simulink model "guidance_formationBreak"  (R2023a)
settings: Solver=ode4  StartTime=0.0  StopTime=10.0  FixedStep=dt  RelTol=1e-3
undefined symbols (not defined in the file): dt, gnc
settings Model: Creator=hugobuurmeijer  LastModifiedBy=hugobuurmeijer

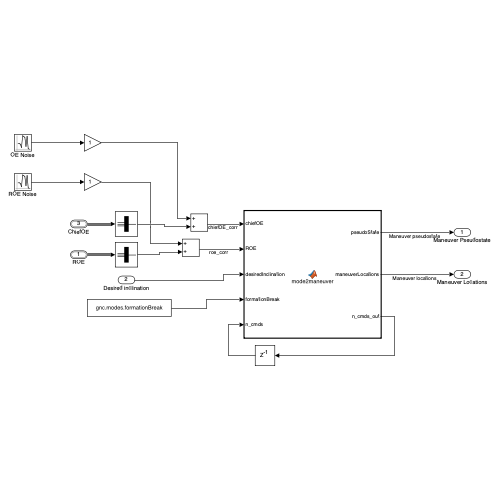
[thumbnail: Simulink's stored preview of the top-level diagram]
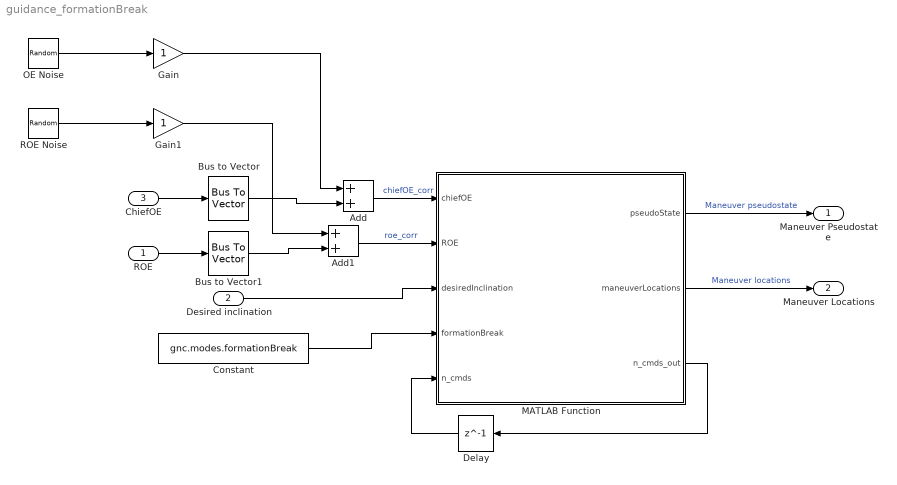
== system guidance_formationBreak ==
  ROE : Inport  OutDataTypeStr=Bus: eccentricSingularROE
  Desired inclination : Inport  Port=2  PortDimensions=2
  ChiefOE : Inport  Port=3  OutDataTypeStr=Bus: meanOrbitElements
  Add : Sum
  Add1 : Sum
  Bus to Vector : BusToVector
  Bus to Vector1 : BusToVector
  Constant : Constant  Value=gnc.modes.formationBreak
  Delay : Delay  DelayLength=1  InitialCondition=0
  Gain : Gain
  Gain1 : Gain
  MATLAB Function : MATLAB Function  TreatAsAtomicUnit=on
  OE Noise : RandomNumber  Mean=zeros(6,1)  Variance=[100,1e-6,1e-6,1e-6,1e-6,1e-46]'  Seed=[1;2;3;4;5;6]  SampleTime=dt
  ROE Noise : RandomNumber  Mean=zeros(6,1)  Variance=1e-12*ones(6,1)  Seed=[1;2;3;4;5;6]  SampleTime=dt
  Maneuver Pseudostate : Outport
  Maneuver Locations : Outport  Port=2
  wires:
  ROE/1 -> Bus to Vector1/1
  Desired inclination/1 -> MATLAB Function/3(desiredInclination)
  MATLAB Function/1(pseudoState) -> Maneuver Pseudostate/1  "Maneuver pseudostate"
  MATLAB Function/2(maneuverLocations) -> Maneuver Locations/1  "Maneuver locations"
  ChiefOE/1 -> Bus to Vector/1
  Bus to Vector/1 -> Add/2
  Bus to Vector1/1 -> Add1/2
  MATLAB Function/3(n_cmds_out) -> Delay/1
  Delay/1 -> MATLAB Function/5(n_cmds)
  Constant/1 -> MATLAB Function/4(formationBreak)
  ROE Noise/1 -> Gain1/1
  Add/1 -> MATLAB Function/1(chiefOE)  "chiefOE_corr"
  OE Noise/1 -> Gain/1
  Add1/1 -> MATLAB Function/2(ROE)  "roe_corr"
  Gain/1 -> Add/1
  Gain1/1 -> Add1/1

== matlab function guidance_formationBreak/MATLAB Function ==
  data: chiefOE input; pseudoState output; ROE input; desiredInclination input; formationBreak input; maneuverLocations output [..69]; n_cmds input; n_cmds_out output
function [pseudoState, maneuverLocations, n_cmds_out] = mode2maneuver(chiefOE, ROE, desiredInclination,formationBreak, n_cmds )

[pseudoState, maneuverLocations,n_cmds_out] = mode2maneuver(chiefOE, ROE, desiredInclination,n_cmds, formationBreak);

end
